simulink model "corner_detector"  (R2024a)
settings: Solver=VariableStepAuto  StartTime=0.0  StopTime=10.0  RelTol=1e-3
undefined symbols (not defined in the file or in its folder): fspecial
libraries: visionanalysis x1, visiontextngfix x1
settings Model: Creator=kosti  LastModifiedBy=kosti

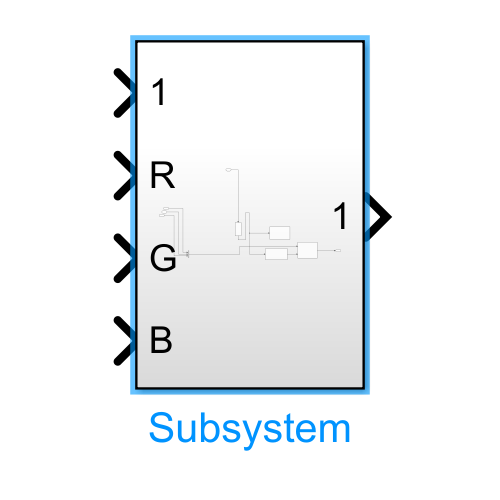
[thumbnail: Simulink's stored preview of the top-level diagram]
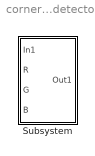
== system corner_detector ==
  Subsystem : Subsystem

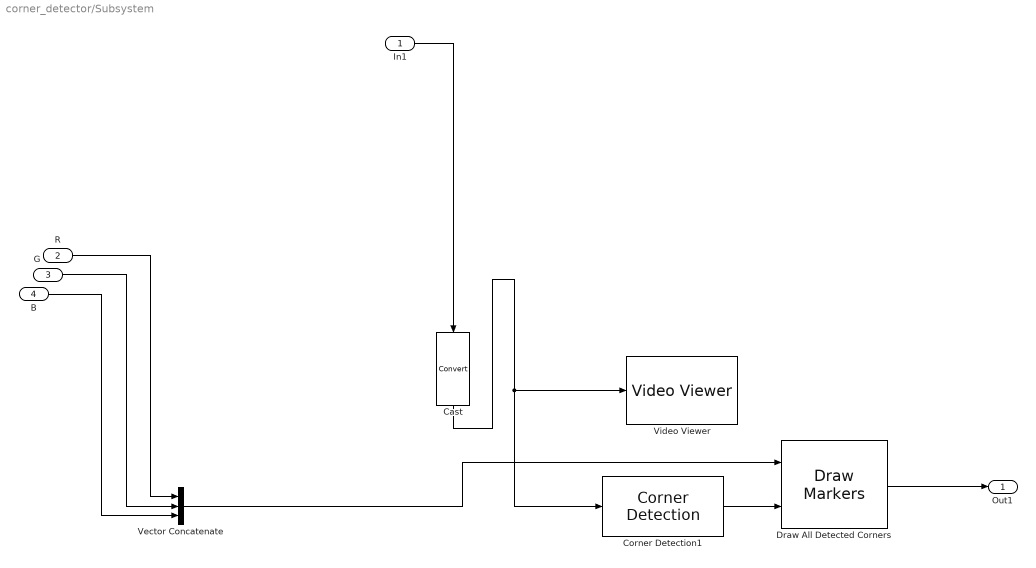
== system corner_detector/Subsystem ==
  In1 : Inport
  R : Inport  Port=2
  G : Inport  Port=3
  B : Inport  Port=4
  Cast : DataTypeConversion  SaturateOnIntegerOverflow=off  RndMeth=Floor
  Corner Detection1 : visionanalysis/Corner Detection  method=Harris corner detection (Harris & Stephens)  factor=0.04  filter=fspecial('gaussian', [1 9], 3)  thrInten=0.1  thrAngle=157.5  output=Obsolete9b  outputInUse=Corner location  maxNum=4  thrMetric=0.0005  neighborSize=[11 11]  isOutVarDim=on  roundingMode=Floor  overflowMode=off  firstCoeffMode=Specify word length  firstCoeffWordLength=16  firstCoeffFracLength=16  prodOutputMode=Binary point scaling  prodOutputWordLength=32  prodOutputFracLength=0  accumMode=Binary point scaling  accumWordLength=32  accumFracLength=0  memoryMode=Binary point scaling  memoryWordLength=32  memoryFracLength=0
  Draw All Detected Corners : visiontextngfix/Draw Markers  shape=Circle  size=9  fill=on  fillClrSource=Specify via dialog  display=User-specified value  intensity=200  color=[250 0 0]  opacity=0.6  viewport=Entire image  antialiasing=off  inType=Obsolete  imagePorts=One multidimensional signal  roundingMode=Floor  overflowMode=off  memoryMode=Specify word length  memoryWordLength=16  memoryFracLength=15  prodOutputMode=Binary point scaling  prodOutputWordLength=32  prodOutputFracLength=14
  Vector Concatenate : Concatenate  NumInputs=3  Mode=Multidimensional array  ConcatenateDimension=3
  Video Viewer : VideoViewer  FigPos=[559 583 418 304]
  Out1 : Outport
  wires:
  Draw All Detected Corners/1 -> Out1/1
  Cast/1 -> Corner Detection1/1, Video Viewer/1
  Vector Concatenate/1 -> Draw All Detected Corners/1
  Corner Detection1/1 -> Draw All Detected Corners/2
  R/1 -> Vector Concatenate/1
  B/1 -> Vector Concatenate/3
  G/1 -> Vector Concatenate/2
  In1/1 -> Cast/1
